simulink model "untitled"  (R2024b)
settings: Solver=VariableStepAuto  StartTime=0.0  StopTime=10  RelTol=1e-3
settings Model: Creator=tarek m eid  LastModifiedBy=tarek m eid

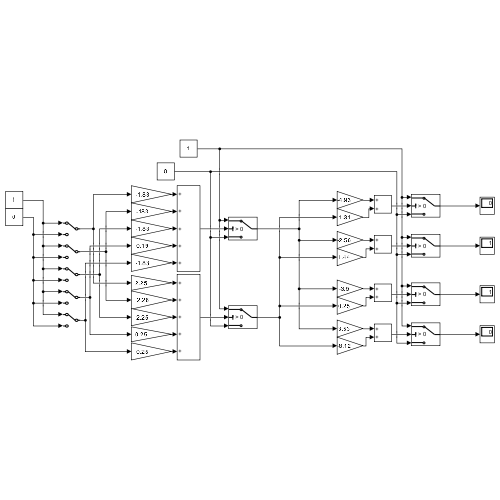
[thumbnail: Simulink's stored preview of the top-level diagram]
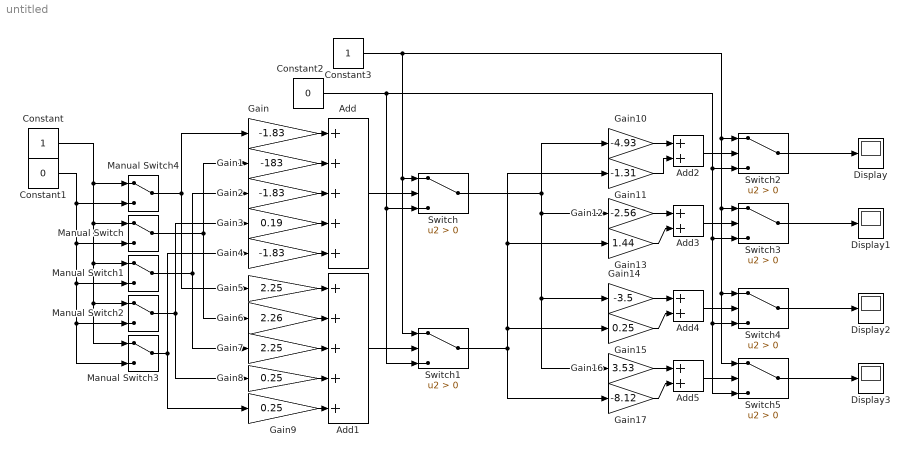
== system untitled ==
  Add : Sum  Inputs=+++++
  Add1 : Sum  Inputs=+++++
  Add{2..5} (4 alike) : Sum
  Constant : Constant
  Constant1 : Constant  Value=0
  Constant2 : Constant  Value=0
  Constant3 : Constant
  Display{,1..3} (4 alike) : Display
  Gain : Gain  Gain=-1.83
  Gain1 : Gain  Gain=-183
  Gain10 : Gain  Gain=-4.93
  Gain11 : Gain  Gain=-1.31
  Gain12 : Gain  Gain=-2.56
  Gain13 : Gain  Gain=1.44
  Gain14 : Gain  Gain=-3.5
  Gain15 : Gain  Gain=0.25
  Gain16 : Gain  Gain=3.53
  Gain17 : Gain  Gain=-8.12
  Gain2 : Gain  Gain=-1.83
  Gain3 : Gain  Gain=0.19
  Gain4 : Gain  Gain=-1.83
  Gain5 : Gain  Gain=2.25
  Gain6 : Gain  Gain=2.26
  Gain7 : Gain  Gain=2.25
  Gain8 : Gain  Gain=0.25
  Gain9 : Gain  Gain=0.25
  Manual Switch{,1..4} (5 alike) : ManualSwitch
  Switch{,1..5} (6 alike) : Switch  Criteria=u2 > Threshold  SaturateOnIntegerOverflow=off  InputSameDT=off
  wires:
  Constant/1 -> Manual Switch3/1, Manual Switch2/1, Manual Switch1/1, Manual Switch/1, Manual Switch4/1
  Constant1/1 -> Manual Switch3/2, Manual Switch2/2, Manual Switch1/2, Manual Switch/2, Manual Switch4/2
  Manual Switch/1 -> Gain1/1, Gain6/1
  Manual Switch4/1 -> Gain/1, Gain5/1
  Manual Switch1/1 -> Gain2/1, Gain7/1
  Manual Switch2/1 -> Gain3/1, Gain8/1
  Manual Switch3/1 -> Gain4/1, Gain9/1
  Gain4/1 -> Add/5
  Gain3/1 -> Add/4
  Gain2/1 -> Add/3
  Gain1/1 -> Add/2
  Gain/1 -> Add/1
  Gain5/1 -> Add1/1
  Gain6/1 -> Add1/2
  Gain7/1 -> Add1/3
  Gain8/1 -> Add1/4
  Gain9/1 -> Add1/5
  Add/1 -> Switch/2
  Add1/1 -> Switch1/2
  Switch/1 -> Gain10/1, Gain16/1, Gain14/1, Gain12/1
  Switch1/1 -> Gain11/1, Gain13/1, Gain15/1, Gain17/1
  Add2/1 -> Switch2/2
  Gain10/1 -> Add2/1
  Gain11/1 -> Add2/2
  Add3/1 -> Switch3/2
  Add4/1 -> Switch4/2
  Add5/1 -> Switch5/2
  Gain12/1 -> Add3/1
  Gain14/1 -> Add4/1
  Gain15/1 -> Add4/2
  Gain13/1 -> Add3/2
  Gain16/1 -> Add5/1
  Gain17/1 -> Add5/2
  Switch2/1 -> Display/1
  Switch3/1 -> Display1/1
  Switch4/1 -> Display2/1
  Switch5/1 -> Display3/1
  Constant3/1 -> Switch5/1, Switch4/1, Switch3/1, Switch2/1, Switch1/1, Switch/1
  Constant2/1 -> Switch5/3, Switch4/3, Switch3/3, Switch2/3, Switch1/3, Switch/3
